simulink model "ATTN"  (R2023a)
settings: Solver=FixedStepAuto  StartTime=0.0  StopTime=40000  RelTol=1e-3
model workspace (MAT data in the model file):
  SampleTime = 0.001
  T_npxls = 4
  T_pupil = 100
  T_whisk = 20
  maxFrame = 3600000
  rewardDuration = 0.05
  targetSide = 1
  toneDuration = 1.5
  trainingStage = 3
  triangleAmplitude = 10
  triangleDuration = 0.1
undefined symbols (not defined in the file or in its folder): Ended, fdesignblkfcn, gcbh, Single
libraries: speedgoatlib_IO191 x5
(part 1 of 3)
settings Model: SimulationMode=external  ExtModeEnableFloating=off  Creator=electro  LastModifiedBy=electro
settings SolverCC: ConcurrentTasks=on  PositivePriorityOrder=on  AutoInsertRateTranBlk=on
settings DataIOCC: SaveFormat=Array
settings OptimizationCC: BlockReduction=off  OptimizeBlockIOStorage=off  EnhancedBackFolding=on  PassReuseOutputArgsThreshold=0  OptimizeBlockOrder=speed  DifferentSizesBufferReuse=on
settings DebuggingCC: TasksWithSamePriorityMsg=none  ParameterTunabilityLossMsg=error  SFUnexpectedBacktrackingDiag=warning  SFNoUnconditionalDefaultTransitionDiag=warning
settings HardwareCC: ProdBitPerLong=64  ProdLongLongMode=on  ProdHWDeviceType=Intel->x86-64 (Linux 64)
settings SFSimCC: SimUserIncludeDirs="\"/usr/local/MATLAB/R2023a/toolbox/slrealtime/target/kernel/dist/include/verify\""  MATLABDynamicMemAlloc=off
settings RTWCC: Description=Simulink Real-Time  SystemTargetFile=slrealtime.tlc  TemplateMakefile=slrealtime_default_tmf  GenerateReport=on  RTWVerbose=off  CustomInclude=/usr/local/MATLAB/R2023a/toolbox/slrealtime/target/kernel/dist/include,  Toolchain=Simulink Real-Time Toolchain  BuildConfiguration=Faster Runs  CodeExecutionProfiling=on  TargetLang=C++
settings CodeAppCC: ForceParamTrailComments=on  OperatorAnnotations=on  EnableCustomComments=on

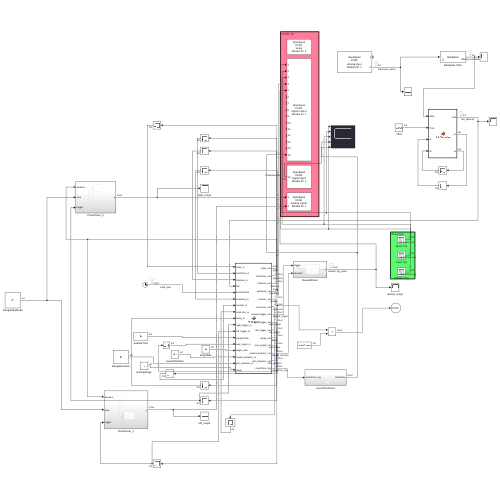
[thumbnail: Simulink's stored preview of the top-level diagram]
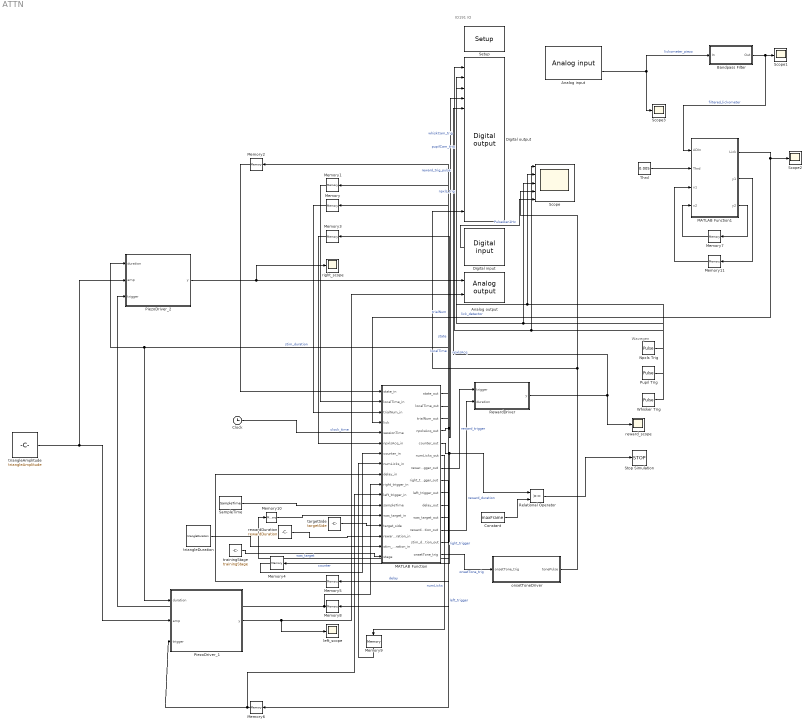
== system ATTN ==
  note: IO191 IO
  note: Wavegen
  "Analog input " : speedgoatlib_IO191/Analog input   parModuleId=1  parSampleTime=-1  parPciSlot=-1  parAdcChannels=[1 2]  parAdcMode=2  parAdcRanges=[3 3]  parAdcRate=100000  parAdcInitValues=[0 0]  parAdcResets=[1 1]
      settings: SourceProductName=Simulink Real-Time: Speedgoat I/O Blockset
  "Analog output " : speedgoatlib_IO191/Analog output   parModuleId=1  parSampleTime=-1  parPciSlot=-1  parDacChannels=[1 3]  parModuleType=1  parDacRanges=[4 4]  parDacInitValues=[0 0]  parDacResets=[1 1]
      settings: SourceProductName=Simulink Real-Time: Speedgoat I/O Blockset
  Bandpass Filter : Subsystem  DialogController=fdesignblkfcn  InitFcn=fdesignblkfcn(gcbh, {'InitFcn'});  mask(Bandpass Filter){}
      mask help: dsp:DSPFilterDesignBlockDialog:BandpassFdesign_MaskDesc
      settings: CopyFcn=fdesignblkfcn(gcbh, {'CopyFcn'});
      mask Help: helpview(mapfilelocation('dsp'), 'dspbandpassfilter');
      mask Display: disp('Bandpass');
  Clock : Clock
      settings: Decimation=1000
  Constant : Constant  Value=maxFrame  VectorParams1D=off  SampleTime=SampleTime
  "Digital input " : speedgoatlib_IO191/Digital input   parModuleId=1  parSampleTime=SampleTime  parPciSlot=-1  parDiChannels=14
      settings: SourceProductName=Simulink Real-Time: Speedgoat I/O Blockset
  "Digital output " : speedgoatlib_IO191/Digital output   parModuleId=1  parSampleTime=0.001  parPciSlot=-1  parDoChannels=[1 2 3 4 5 6 7 8 9 10 11 12 13 15 16]  parDoInitValues=[0 0 0 0 0 0 0 0 0 0 0 0 0 0 0]  parDoResets=[1 1 1 1 1 1 1 1 1 1 1 1 1 1 1]
      settings: SourceProductName=Simulink Real-Time: Speedgoat I/O Blockset
  MATLAB Function : MATLAB Function  TreatAsAtomicUnit=on
  MATLAB Function1 : MATLAB Function  TreatAsAtomicUnit=on
  Memory{,1,5..11} (9 alike) : Memory
  Memory2 : Memory  InitialCondition=1
  Memory3 : Memory  InitialCondition=1
  Memory4 : Memory  InitialCondition=1
  Npxls Trig : DiscretePulseGenerator  Amplitude=2.5  Period=T_npxls  PulseWidth=T_npxls/2  SampleTime=SampleTime
  PiezoDriver_1 : Subsystem
  PiezoDriver_2 : Subsystem
  Pupil Trig : DiscretePulseGenerator  Period=T_pupil  PulseWidth=T_pupil/2  SampleTime=SampleTime
  Relational Operator : RelationalOperator  OutDataTypeStr=boolean  RndMeth=Simplest  InputSameDT=off
  RewardDriver : Subsystem
  SampleTime : Constant  Value=SampleTime  SampleTime=SampleTime
  Scope : Scope  NumInputPorts=5
  Scope1 : Scope
  Scope2 : Scope
  Scope3 : Scope
  "Setup " : speedgoatlib_IO191/Setup   parModuleId=1  parPciSlot=-1  parTriggerSignal=TTL  parAdcChannels=[1 2]  parAdcRanges=[3 3]  parAdcChannel1=on  parAdcChannel2=on  parAdcChannel3=off  parAdcChannel4=off  parAdcChannel5=off  parAdcChannel6=off  parAdcChannel7=off  parAdcChannel8=off  parAdcMode=Single-Ended  parAdcRate=100000  parAdcRange11=+-10.24 V  parAdcRange21=+-24.576 V  parAdcRange12=+-10.24 V  parAdcRange22=+-24.576 V  parAdcRange13=+-10.24 V  parAdcRange23=+-24.576 V  parAdcRange14=+-10.24 V  parAdcRange24=+-24.576 V  parAdcRange15=+-10.24 V  parAdcRange25=+-24.576 V  parAdcRange16=+-10.24 V  parAdcRange26=+-24.576 V  parAdcRange17=+-10.24 V  parAdcRange27=+-24.576 V  parAdcRange18=+-10.24 V  parAdcRange28=+-24.576 V  parDacChannels=[1 3]  parDacChannel1=on  parDacChannel2=off  parDacChannel3=on  parDacChannel4=off  parDacMode=Single-Ended  parDacRanges=[4 4]  parDacInitValues=[0 0]  parDacResets=[1 1]  parDacRange1=+-10 V  parDacInitValue1=0  parDacReset1=on  parDacRange2=+-10 V  parDacInitValue2=0  parDacReset2=on  parDacRange3=+-10 V  parDacInitValue3=0  parDacReset3=on  parDacRange4=+-10 V  parDacInitValue4=0  parDacReset4=on  parDiChannels=14  parDoChannels=[1 2 3 4 5 6 7 8 9 10 11 12 13 15 16]  parDioFirstControl=[1 2 3 4 5 6 8 9]  parDioSecondControl=0  parDioChannel1=Out  parExtra1=I  parExtra2=I  parExtra3=I  parDioChannel2=Out  parDioChannel3=Out  parDioChannel4=Out  parDioChannel5=Out  parDioChannel6=Out  parDioChannel7=In  parDioChannel8=Out  parDioChannel9=Out  parDoInitValues=[0 0 0 0]  parDoResets=[1 1 1 1]  parDoInitValue1=0  parDoReset1=on  parDoInitValue2=0  parDoReset2=on  parDoInitValue3=0  parDoReset3=on  parDoInitValue4=0  parDoReset4=on  parDoInitValue5=0  parDoReset5=on  parDoInitValue6=0  parDoReset6=on  parDoInitValue7=0  parDoReset7=on  parDoInitValue8=0  parDoReset8=on  parDoInitValue9=0  parDoReset9=on  parDoInitValue10=0  parDoReset10=on  parDoInitValue11=0  parDoReset11=on  parDoInitValue12=0  parDoReset12=on  parDoInitValue13=0  parDoReset13=on  parDoInitValue14=0  parDoReset14=on  parDoInitValue15=0  parDoReset15=on  parDoInitValue16=0  parDoReset16=on
      settings: SourceProductName=Simulink Real-Time: Speedgoat I/O Blockset
  Stop Simulation : Stop
  Thrd : Constant  Value=0.005
  Whisker Trig : DiscretePulseGenerator  Period=T_whisk  PulseWidth=T_whisk/2  SampleTime=SampleTime
  left_scope : Scope
  onsetToneDriver : Subsystem
  rewardDuration : Constant  Value=rewardDuration
  reward_scope : Scope
  right_scope : Scope
  targetSide : Constant  Value=targetSide
  trainingStage : Constant  Value=trainingStage
  triangleAmplitude : Constant  Value=triangleAmplitude
  triangleDuration : Constant  Value=triangleDuration
  wires:
  Relational Operator/1 -> Stop Simulation/1
  Constant/1 -> Relational Operator/2
  MATLAB Function/11(was_target_out) -> Memory10/1  "was_target"
  Memory5/1 -> MATLAB Function/9(delay_in)
  Memory1/1 -> MATLAB Function/2(localTime_in)
  Memory10/1 -> MATLAB Function/13(was_target_in)
  Memory4/1 -> MATLAB Function/7(counter_in)
  Memory/1 -> MATLAB Function/3(trialNum_in)
  Memory2/1 -> MATLAB Function/1(state_in)
  Whisker Trig/1 -> "Digital output "/1, Scope/1  "whiskCam_trig"
  Pupil Trig/1 -> Scope/3, "Digital output "/3  "pupilCam_trig"
  Clock/1 -> MATLAB Function/5(sessionTime)  "clock_time"
  Memory9/1 -> MATLAB Function/8(numLicks_in)
  MATLAB Function/4(npxlsAcq_out) -> "Digital output "/4, Memory3/1  "npxlsAcq"
  Memory3/1 -> MATLAB Function/6(npxlsAcq_in)
  MATLAB Function/3(trialNum_out) -> Memory/1  "trialNum"
  Npxls Trig/1 -> "Digital output "/2, Scope/2  "npxls_trig"
  MATLAB Function/2(localTime_out) -> Memory1/1  "localTime"
  SampleTime/1 -> MATLAB Function/12(sampleTime)
  MATLAB Function/1(state_out) -> Memory2/1  "state"
  MATLAB Function/5(counter_out) -> Relational Operator/1, Memory4/1  "counter"
  MATLAB Function/6(numLicks_out) -> Memory9/1  "numLicks"
  MATLAB Function/8(right_trigger_out) -> Memory8/1  "right_trigger"
  MATLAB Function/9(left_trigger_out) -> Memory6/1  "left_trigger"
  MATLAB Function/10(delay_out) -> Memory5/1  "delay"
  "Digital input "/1 -> Scope/5  "PulseGen1Hz"
  targetSide/1 -> MATLAB Function/14(target_side)
  trainingStage/1 -> MATLAB Function/17(stage)
  Memory8/1 -> PiezoDriver_2/3(trigger), MATLAB Function/10(right_trigger_in)
  Memory6/1 -> PiezoDriver_1/3(trigger), MATLAB Function/11(left_trigger_in)
  triangleAmplitude/1 -> PiezoDriver_2/2(amp), PiezoDriver_1/2(amp)
  PiezoDriver_1/1(y) -> left_scope/1, "Analog output "/2
  PiezoDriver_2/1(y) -> "Analog output "/1, right_scope/1
  rewardDuration/1 -> MATLAB Function/15(reward_duration_in)
  RewardDriver/1(y) -> reward_scope/1, "Digital output "/5  "reward_trig_pulse"
  MATLAB Function/7(reward_trigger_out) -> RewardDriver/1(trigger)  "reward_trigger"
  MATLAB Function/12(reward_duration_out) -> RewardDriver/2(duration)  "reward_duration"
  triangleDuration/1 -> MATLAB Function/16(stim_duration_in)
  MATLAB Function/13(stim_duration_out) -> PiezoDriver_1/1(duration), PiezoDriver_2/1(duration)  "stim_duration"
  onsetToneDriver/1(tonePulse) -> Scope/4, "Digital output "/15
  MATLAB Function/14(onsetTone_trig) -> onsetToneDriver/1(onsetTone_trig)  "onsetTone_trig"
  MATLAB Function1/3(y2) -> Memory7/1
  Memory7/1 -> MATLAB Function1/4(x2)
  MATLAB Function1/2(y1) -> Memory11/1
  Memory11/1 -> MATLAB Function1/3(x1)
  Thrd/1 -> MATLAB Function1/2(Thrd)
  "Analog input "/2 -> Bandpass Filter/1(In), Scope3/1  "lickometer_piezo"
  MATLAB Function1/1(Lick) -> Scope2/1, MATLAB Function/4(lick)  "lick_detector"
  Bandpass Filter/1(Out) -> MATLAB Function1/1(ADIn), Scope1/1  "filtered_lickometer"
